simulink model "problem_2"  (R2022b)
settings: Solver=VariableStepAuto  StartTime=0.0  StopTime=0.4  RelTol=1e-3
libraries: simulink x4
settings Model: Creator=Mahadevu Sudheer  LastModifiedBy=Mahadevu Sudheer

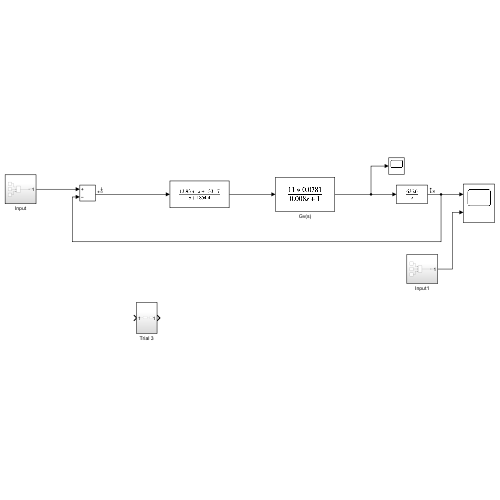
[thumbnail: Simulink's stored preview of the top-level diagram]
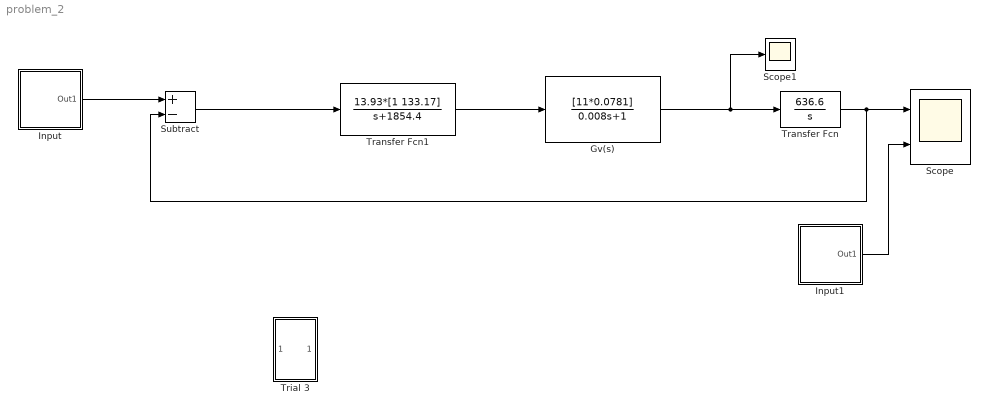
== system problem_2 ==
  Gv(s) : TransferFcn  Numerator=[11*0.0781]  Denominator=[0.008 1]
  Input : Subsystem
  Input1 : Subsystem
  Scope : Scope  NumInputPorts=2
  Scope1 : Scope
  Subtract : Sum  Inputs=+-
  Transfer Fcn : TransferFcn  Numerator=[636.6]  Denominator=[1 0]
  Transfer Fcn1 : TransferFcn  Numerator=13.93*[1 133.17]  Denominator=[1 1854.4]
  Trial 3 : Subsystem
  wires:
  Gv(s)/1 -> Scope1/1, Transfer Fcn/1
  Transfer Fcn/1 -> Scope/1, Subtract/2
  Input/1(Out1) -> Subtract/1
  Subtract/1 -> Transfer Fcn1/1
  Transfer Fcn1/1 -> Gv(s)/1
  Input1/1(Out1) -> Scope/2

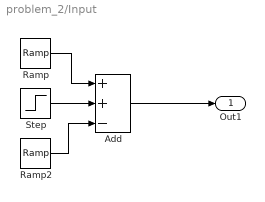
== system problem_2/Input ==
  Add : Sum  Inputs=++-
  Ramp : simulink/Sources/Ramp  slope=10000  start=0  InitialOutput=0  VectorParams1D=off
  Ramp2 : simulink/Sources/Ramp  slope=10000  start=0.25  InitialOutput=0  VectorParams1D=off
  Step : Step  Time=0.25  After=0  SampleTime=0
  Out1 : Outport
  wires:
  Ramp2/1 -> Add/3
  Add/1 -> Out1/1
  Ramp/1 -> Add/1
  Step/1 -> Add/2

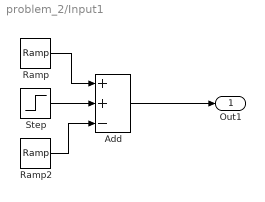
== system problem_2/Input1 ==
  Add : Sum  Inputs=++-
  Ramp : simulink/Sources/Ramp  slope=10000  start=0  InitialOutput=0  VectorParams1D=off
  Ramp2 : simulink/Sources/Ramp  slope=10000  start=0.25  InitialOutput=0  VectorParams1D=off
  Step : Step  Time=0.25  After=0  SampleTime=0
  Out1 : Outport
  wires:
  Ramp2/1 -> Add/3
  Add/1 -> Out1/1
  Ramp/1 -> Add/1
  Step/1 -> Add/2

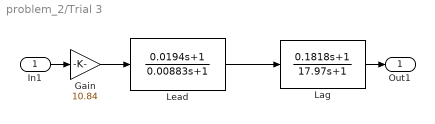
== system problem_2/Trial 3 ==
  In1 : Inport
  Gain : Gain  Gain=10.84
  "Lag " : TransferFcn  Numerator=[0.1818 1]  Denominator=[17.97 1]
  Lead : TransferFcn  Numerator=[0.0194 1]  Denominator=[0.00883 1]
  Out1 : Outport
  wires:
  Lead/1 -> "Lag "/1
  Gain/1 -> Lead/1
  In1/1 -> Gain/1
  "Lag "/1 -> Out1/1
